simulink model "adcs_sim_main2"  (R2017b)
settings: Solver=FixedStepAuto  StartTime=0.0  StopTime=360  RelTol=1e-3  EnableMultiTasking=on
InitFcn:
  | %sim_init
StopFcn:
  | %% Extract States
  | %states = logsout.getElement('states').Values;
  | %sc_quat = states.quaternion;
  | %omega_radps = states.body_rates_radps;
  | %pos_eci_km = states.position_eci_km;
  | %vel_eci_kmps = states.velocity_eci_kmps;
  | 
  | %% Extract Actuator measurements
  | %act_meas = logsout.getElement('act_meas').Values;
  | 
  | %% Extract Commands
  | %cmds = logsout.getElement('commands').Values;
  | %MT_dv = cmds.MT_dv;
  | 
  | %% Extract sensor processing output
  | %sp2fsw = logsout.getElement('sp2fsw').Values;
  | %mag_meas = sp2fsw.mag_vec_body_T;
  | 
  | %% Extract B-dot tumble status
  | %tumble = logsout.getElement('tumble').Values;
  | %tumble_t = logsout.getElement('tumble').Time;
libraries: actuators_lib x1, dynamics_lib x1, environment_lib x1, sldrtlib x1, sensors_lib x1, aerolibanimutils x1
settings Model: Creator=bbarz_000  LastModifiedBy=SatLab
settings SolverCC: AutoInsertRateTranBlk=on
settings DataIOCC: SaveOutput=off
settings OptimizationCC: DefaultParameterBehavior=Inlined  UseDivisionForNetSlopeComputation=on  UseFloatMulNetSlope=on  InlineInvariantSignals=on  PassReuseOutputArgsAs=Individual arguments  ZeroExternalMemoryAtStartup=off  ZeroInternalMemoryAtStartup=off  NoFixptDivByZeroProtection=on  EfficientFloat2IntCast=on  LifeSpan=1
settings DebuggingCC: ParameterTunabilityLossMsg=error  SFUnexpectedBacktrackingDiag=warning  SFNoUnconditionalDefaultTransitionDiag=warning  SFExecutionAtInitializationDiag=none
settings HardwareCC: ProdBitPerInt=16  ProdBitPerPointer=16  ProdBitPerSizeT=16  ProdBitPerPtrDiffT=16  ProdLargestAtomicFloat=None  ProdWordSize=16  ProdHWDeviceType=Texas Instruments->MSP430
settings SFSimCC: MATLABDynamicMemAlloc=off
settings RTWCC: SystemTargetFile=ert.tlc  GenCodeOnly=on  PackageGeneratedCodeAndArtifacts=on  TemplateMakefile=ert_default_tmf  GenerateReport=on  Toolchain=Clang v3.1 | gmake (64-bit Mac)  IncludeHyperlinkInReport=on  LaunchReport=on  GenerateTraceInfo=on  GenerateTraceReport=on  GenerateTraceReportSl=on  GenerateTraceReportSf=on  GenerateTraceReportEml=on  GenerateCodeMetricsReport=on
settings CodeAppCC: ForceParamTrailComments=on  IgnoreCustomStorageClasses=off  OperatorAnnotations=on  SimulinkDataObjDesc=on  SFDataObjDesc=on  MATLABFcnDesc=on  CustomSymbolStrGlobalVar=rt$N$M  CustomSymbolStrType=$N$M  CustomSymbolStrFcn=$N$M$F  CustomSymbolStrMacro=$N$M  InsertBlockDesc=on  StateflowObjectComments=on  MATLABSourceComments=on
settings ERTTargetCC: MultiwordLength=2048  GenerateSampleERTMain=on  CombineSignalStateStructs=on  SupportComplex=off  SupportContinuousTime=on  SupportNonInlinedSFcns=on  InlinedParameterPlacement=NonHierarchical  ERTCustomFileTemplate=example_file_process.tlc  ERTFilePackagingFormat=CompactWithDataFile
settings ConfigComp: CovMetricSettings=dw  CovHtmlReporting=on  CovSaveCumulativeToWorkspaceVar=on  CovSaveSingleToWorkspaceVar=on  CovExternalEMLEnable=off
settings SimscapeCC: SimscapeNormalizeSystem=off

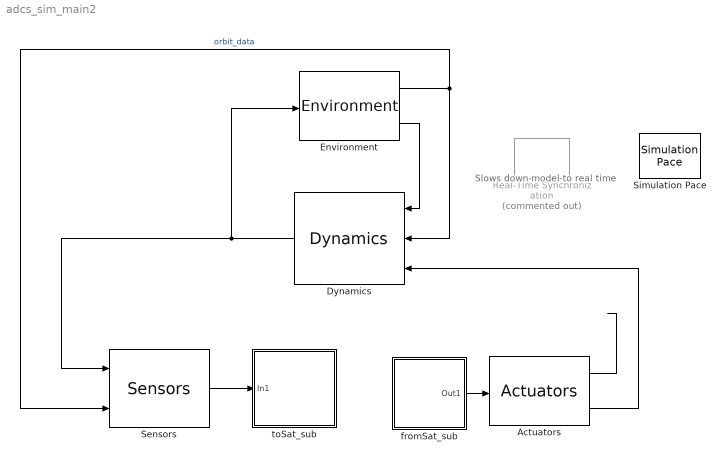
== system adcs_sim_main2 ==
  note: Slows down model to real time
  Actuators : actuators_lib/Actuators
      link override Bus Selector: OutputSignals=MT_dv
  Dynamics : dynamics_lib/Dynamics
  Environment : environment_lib/Environment
  Real-Time Synchronization : sldrtlib/Real-Time Synchronization  Commented=on  SampleTime=0.1  MaxMissedTicks=10  ShowMissedTicks=off  YieldWhenWaiting=off
  Sensors : sensors_lib/Sensors
  Simulation Pace : aerolibanimutils/Simulation Pace  SimulationPace=1  SleepMode=MATLAB Thread  OutputPaceError=off  SampleTime=1/30
  fromSat_sub : Subsystem
  toSat_sub : Subsystem
  wires:
  Dynamics/1 -> Environment/1, Sensors/1
  Environment/1 -> Sensors/2, Dynamics/2  "orbit_data"
  Actuators/2 -> Dynamics/3
  Actuators/1 -> ?
  Environment/2 -> Dynamics/1
  Sensors/1 -> toSat_sub/1(In1)
  fromSat_sub/1(Out1) -> Actuators/1

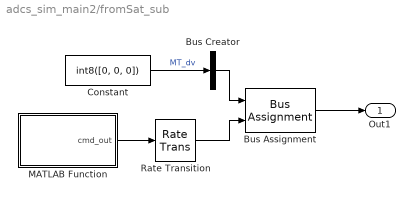
== system adcs_sim_main2/fromSat_sub ==
  Bus Assignment : BusAssignment  AssignedSignals=MT_dv
  Bus Creator : BusCreator  Inputs=1
  Constant : Constant  Value=int8([0, 0, 0])  VectorParams1D=off  OutDataTypeStr=int8
  MATLAB Function : MATLAB Function  TreatAsAtomicUnit=on
  Rate Transition : RateTransition
  Out1 : Outport
  wires:
  Bus Assignment/1 -> Out1/1
  Bus Creator/1 -> Bus Assignment/1
  Constant/1 -> Bus Creator/1  "MT_dv"
  MATLAB Function/1(cmd_out) -> Rate Transition/1
  Rate Transition/1 -> Bus Assignment/2

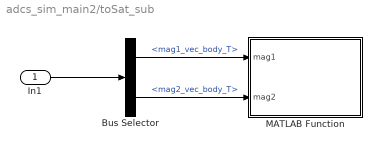
== system adcs_sim_main2/toSat_sub ==
  In1 : Inport
  Bus Selector : BusSelector  OutputSignals=mag1_vec_body_T,mag2_vec_body_T
  MATLAB Function : MATLAB Function  TreatAsAtomicUnit=on
  wires:
  In1/1 -> Bus Selector/1
  Bus Selector/1 -> MATLAB Function/1(mag1)  "<mag1_vec_body_T>"
  Bus Selector/2 -> MATLAB Function/2(mag2)  "<mag2_vec_body_T>"

== matlab function adcs_sim_main2/toSat_sub/MATLAB Function ==
  data: mag1 input; mag2 input
 function toSat(mag1, mag2)
%{
Puts data on BDOT board via Aardvark for use in HIL sim
Each parameter contains x,y,z data and a valid bit for the corresponding magnetometer
Data is in milliteslas.
%}

% ToDo: Figure out data conversion 

% Implemented a persistent counter that we can compare against
% system time in order to slow down the Aardvark library calls to something
% like 5-10Hz 

%% Extrinsic declarations to bypass code generation in simulink
coder.extrinsic('libisloaded', 'loadlibrary', 'calllib', 'exist', 'now', ...
                'datevec', 'num2str', 'strcat');

%% Persistent Variables

persistent ptime; % For use in timing Aardvark library calls
if isempty(ptime)
    tmp = datevec(now);
    ptime = tmp(6);
    ptime
end

persistent hdev;
if isempty(hdev)
    hdev = 0;
    hdev
end

persistent iter_count;
if isempty(iter_count)
    iter_count = 1;
    iter_count
end

% The time condition looks like this: 
% If ctime >= ptime + 0.2 (or something equivalent to get 5Hz)
%   then do things

%% Setting up Aardvark 

% Configures Aardvark to listen as a slave, using native API wrapper
slaveaddr = hex2dec('1E');
outstr = zeros(6);

% if ~exist('hdev', 'var')
%     hdev = 0; % extrinsic stuff
% end
 
lib = 'aardvark';
libhdr = 'aardvark.h';

% to be run only once
if ~libisloaded(lib)
    "Prepping aardvark"
    loadlibrary(lib, libhdr);
    
    hport = 0;
    calllib(lib, 'c_aa_close', hport);
    
    % opens the aardvark
    hdev = calllib(lib, 'c_aa_open', hport); 
    if (hdev < 0)
        error('Unable to open port 0.');
    end
    
    % sets Aardvark slave response
    calllib(lib, 'c_aa_i2c_slave_set_response', hdev, length(outstr), outstr);
    % configures I2C pullup resisters ( 0 -> None )
    calllib(lib, 'c_aa_i2c_pullup', hdev, 0);
    % enables Aardvark as slave
    calllib(lib, 'c_aa_i2c_slave_enable', hdev, slaveaddr, 0, 0);
    "Aardvark prepped"
end

% Time check
ctime = datevec(now);
ptime_doub = 0.0; % matlab type stuff
ptime_doub = ptime;
ctime_doub = 0.0;
ctime_doub = ctime(6);

results = 0;

% if ctime_doub >= ptime_doub + 1
    iter_count = iter_count + 1;
    %% Convert magnetometer data for sending to Aardvark
    
    % convert from milliteslas to gauss:
    mag1 = 10000 * mag1;
%     mag2 = 10000 * mag2;
%     set magnetometer gain. This should probably just be constant:
    gain = 1370; % LSB / gauss

    % now convert these values in gauss, to a 12 bit value corresponding to strength
    mag1_bits = int16( mag1 * gain );

    % (Mag2 UNUSED)
    % mag2_bits = int16( mag2 * gain );

    % get the most/least significant bit:
    % Mag1
    mag1_x_lsb = uint8(bi2de(bitget( mag1_bits(1), 1:8 )));
    mag1_x_msb = uint8(bi2de(bitget( mag1_bits(1), 9:16 )));

    mag1_y_lsb = uint8(bi2de(bitget( mag1_bits(2), 1:8 )));
    mag1_y_msb = uint8(bi2de(bitget( mag1_bits(2), 9:16 )));

    mag1_z_lsb = uint8(bi2de(bitget( mag1_bits(3), 1:8 )));
    mag1_z_msb = uint8(bi2de(bitget( mag1_bits(3), 9:16 )));

    % Mag2 (UNUSED)
    % mag2_x_lsb = bitget( mag2_bits(1), 1:8 );
    % mag2_x_msb = bitget( mag2_bits(1), 9:16 );
    % 
    % mag2_y_lsb = bitget( mag2_bits(2), 1:8 );
    % mag2_y_msb = bitget( mag2_bits(2), 9:16 );
    % 
    % mag2_z_lsb = bitget( mag2_bits(3), 1:8 );
    % mag2_z_msb = bitget( mag2_bits(3), 9:16 );

    %% Prepping Data

    % outstr takes xMagMsb, Lsb, zMagMsb, Lsb, yMagMsb, Lsb

    % Next line from AardvarkExperiments.m :
%     outstr = [xMagMsb(index) xMagLsb(index) zMagMsb(index) zMagLsb(index) yMagMsb(index) yMagLsb(index)];
   
    outstr = [mag1_x_msb, mag1_x_lsb, mag1_z_msb, mag1_z_lsb, mag1_y_msb, mag1_y_lsb];
%     outstr = uint8(outstr);
%     outstr = uint8([220 (138+20*floor(sin(ptime_doub))) 0 (210+20*floor(sin(ptime_doub))) 0 210]);

    %% Sending Data
    
%     outstr
%     class(outstr)
%     length(outstr)
%     hdev
    calllib(lib, 'c_aa_i2c_slave_set_response', hdev, length(outstr), outstr);

    % calllib(lib, 'c_aa_spi_slave_enable');
    
    % update prev time to curr time
    ptime = ctime(6);
% end

end

== matlab function adcs_sim_main2/fromSat_sub/MATLAB Function ==
  data: cmd_out output
function cmd_out = fcn()

cmd_out = int8([0, 0, 0]);

% TODO: Switch to asynch reads to try and fix the synchronicity error

%% Extrinsic declarations to bypass code generation in simulink
coder.extrinsic('serial');

%% Persistent Variables

persistent s cmd_persistent;
if isempty(s)
    s = serial('COM8');
    s.InputBufferSize = 100;
    fopen(s);
    s
    s.ReadAsyncMode = 'continuous';
end

% Persists between method calls in case of no update in data
if isempty(cmd_persistent)
    cmd_persistent = int8([0, 0, 0]);
    cmd_persistent
end

%% Reading shit hell yeah

mtq_packet_length = 6;
% length of packet meta data (3 bytes)
packet_meta_length = 3;

% data packet header of mtq commands
mtq_header = [252, 6, 126];

out = unicode2native(fscanf(s));
header_indices = strfind(out, mtq_header);
if ~isempty(header_indices)
    header_index = header_indices(1);
    if header_index + mtq_packet_length < length(out)
        cmd_persistent(1) = out(header_index + packet_meta_length);
        cmd_persistent(2) = out(header_index + packet_meta_length + 1);
        cmd_persistent(3) = out(header_index + packet_meta_length + 2);
    end  
end

cmd_out = cmd_persistent;
cmd_out

end
